simulink model "ballbeam_start"  (R2020b)
settings: Solver=ode4  StartTime=0.0  StopTime=inf  FixedStep=0.002  RelTol=1e-3
model workspace (MAT data in the model file):
  Kc = 14.8792
  Wf = 31.4
  z = 4.0159
undefined symbols (not defined in the file or in its folder): HIL, qc_get_step_size
libraries: quarc_library x3, simulink_extras x1
settings Model: ExtModeTrigDuration=12500  Creator=MLevis  LastModifiedBy=kevin
settings DataIOCC: ReturnWorkspaceOutputs=off
settings DebuggingCC: UnderspecifiedInitializationDetection=Classic  MergeDetectMultiDrivingBlocksExec=none
settings ModelReferenceCC: PropagateSignalLabelsOutOfModel=off
settings SFSimCC: CustomCodeUndefinedFunction=UseInterfaceOnly

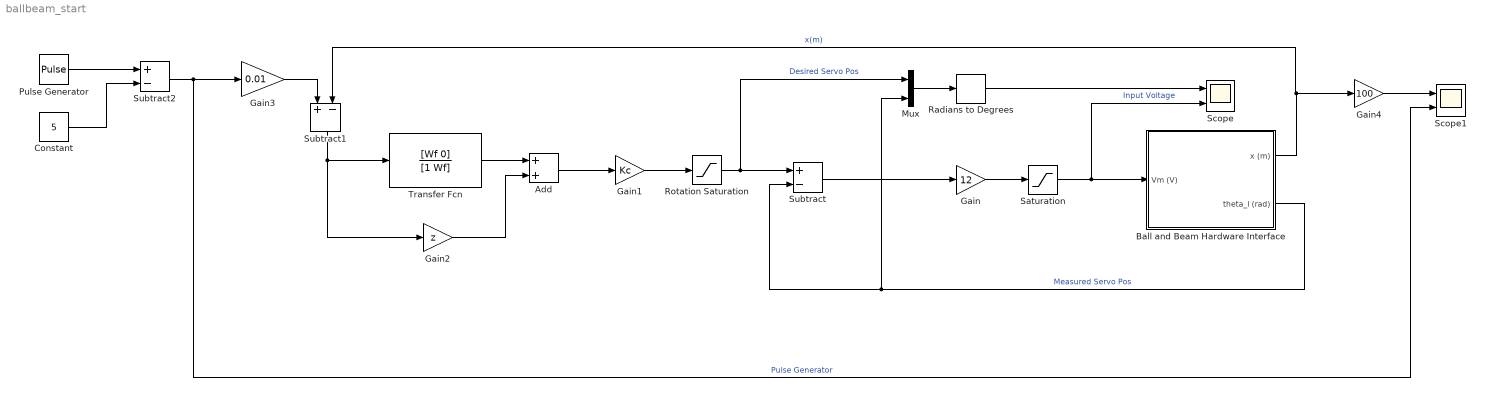
== system ballbeam_start ==
  Add : Sum
  Ball and Beam Hardware Interface : Subsystem
  Constant : Constant  Value=5
  Gain : Gain  Gain=12
  Gain1 : Gain  Gain=Kc
  Gain2 : Gain  Gain=z
  Gain3 : Gain  Gain=0.01
  Gain4 : Gain  Gain=100
  Mux : Mux  Inputs=2
  Pulse Generator : DiscretePulseGenerator  PulseType=Time based  Amplitude=10  Period=10  PulseWidth=50
  Radians to Degrees : simulink_extras/Transformations/Radians to Degrees
  Rotation Saturation : Saturate  UpperLimit=56  LowerLimit=-56
  Saturation : Saturate  UpperLimit=10  LowerLimit=-10
  Scope : Scope  NumInputPorts=2
  Scope1 : Scope  NumInputPorts=2
  Subtract : Sum  Inputs=+-
  Subtract1 : Sum  Inputs=+-
  Subtract2 : Sum  Inputs=+-
  Transfer Fcn : TransferFcn  Numerator=[Wf 0]  Denominator=[1 Wf]
  wires:
  Saturation/1 -> Scope/2, Ball and Beam Hardware Interface/1(Vm (V))  "Input Voltage"
  Gain/1 -> Saturation/1
  Ball and Beam Hardware Interface/2(theta_l (rad)) -> Mux/2, Subtract/2  "Measured Servo Pos"
  Rotation Saturation/1 -> Mux/1, Subtract/1  "Desired Servo Pos"
  Mux/1 -> Radians to Degrees/1
  Radians to Degrees/1 -> Scope/1
  Gain1/1 -> Rotation Saturation/1
  Add/1 -> Gain1/1
  Transfer Fcn/1 -> Add/1
  Gain2/1 -> Add/2
  Subtract1/1 -> Gain2/1, Transfer Fcn/1
  Ball and Beam Hardware Interface/1(x (m)) -> Gain4/1, Subtract1/2  "x(m)"
  Gain3/1 -> Subtract1/1
  Gain4/1 -> Scope1/1
  Constant/1 -> Subtract2/2
  Pulse Generator/1 -> Subtract2/1
  Subtract2/1 -> Scope1/2, Gain3/1  "Pulse Generator"
  Subtract/1 -> Gain/1

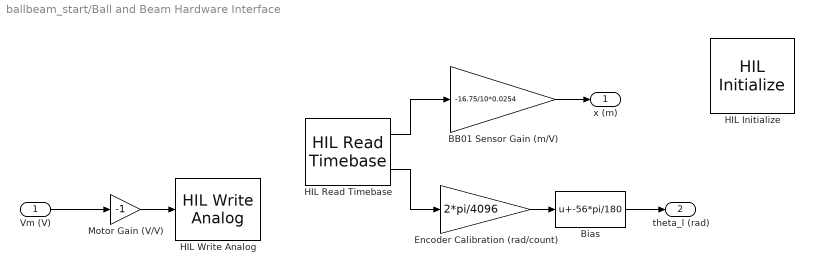
== system ballbeam_start/Ball and Beam Hardware Interface ==
  Vm (V) : Inport
  BB01 Sensor Gain (m/V) : Gain  Gain=-16.75/10*0.0254
  Bias : Bias  Bias=-56*pi/180
  Encoder Calibration (rad/count) : Gain  Gain=2*pi/4096  SaturateOnIntegerOverflow=on  OutDataTypeStr=Inherit: Same as input  ParamDataTypeStr=Inherit: Same as input
  HIL Initialize : quarc_library/Data Acquisition/Generic/Configuration/HIL Initialize  object_name=HIL-1  board_type=q8_usb  board_number=0@tcpip://localhost:18942  board_options=""  exclusive=off  active=on  hardware_clocks=[0:2]  clock_modes=[]  initial_clock_frequencies=[]  set_clock_params_at_start=off  set_clock_params_at_switch_in=off  set_clock_frequencies_at_start=off  set_clock_frequencies_at_switch_in=off  analog_input_channels=[0:7]  analog_input_configurations=[]  analog_input_maximums=10  analog_input_minimums=-10  set_analog_input_params_at_start=on  set_analog_input_params_at_switch_in=off  analog_output_channels=[0:7]  analog_output_maximums=10  analog_output_minimums=-10  initial_analog_outputs=[0]  final_analog_outputs=[0]  watchdog_analog_outputs=0  set_analog_output_params_at_start=on  set_analog_output_params_at_switch_in=off  set_analog_outputs_at_start=on  set_analog_outputs_at_switch_in=off  set_analog_outputs_at_terminate=on  set_analog_outputs_at_switch_out=off  set_analog_outputs_on_watchdog=off  digital_input_channels=[]  digital_output_channels=[0:7]  digital_output_configuration=[]  initial_digital_outputs=[0]  final_digital_outputs=[0]  watchdog_digital_outputs=[0]  set_digital_output_params_at_start=off  set_digital_output_params_at_switch_in=off  set_digital_outputs_at_start=on  set_digital_outputs_at_switch_in=off  set_digital_outputs_at_terminate=on  set_digital_outputs_at_switch_out=off  set_digital_outputs_on_watchdog=off  encoder_channels=[0:7]  quadrature=[4]  encoder_filter_frequency=[]  initial_encoder_counts=[0]  set_encoder_params_at_start=on  set_encoder_params_at_switch_in=off  set_encoder_counts_at_start=on  set_encoder_counts_at_switch_in=off  pwm_channels=[0:7]  pwm_modes=0  pwm_frequency=99.532799999999995e6/4095  pwm_configuration=[0]  pwm_alignment=[0]  pwm_polarity=[1]  pwm_leading_deadband=[0]  pwm_trailing_deadband=[0]  initial_pwm_outputs=[0]  final_pwm_outputs=[0]  watchdog_pwm_outputs=[0]  set_pwm_params_at_start=on  set_pwm_params_at_switch_in=off  set_pwm_outputs_at_start=on  set_pwm_outputs_at_switch_in=off  set_pwm_outputs_at_terminate=on  set_pwm_outputs_at_switch_out=off  set_pwm_outputs_on_watchdog=off  other_output_channels=[]  initial_other_outputs=[]  final_other_outputs=[]  watchdog_other_outputs=[]  set_other_outputs_at_start=off  set_other_outputs_at_switch_in=off  set_other_outputs_at_terminate=off  set_other_outputs_at_switch_out=off  set_other_outputs_on_watchdog=off
  HIL Read Timebase : quarc_library/Data Acquisition/Generic/Timebases/HIL Read Timebase  object_name=HIL-1  clock=0  analog_channels=0  encoder_channels=[0]  digital_channels=[]  other_channels=[]  active=on  vector_output=off  data_type_mode=Inherit via back propagation  encoder_data_type=double  digital_data_type=boolean  overflow_mode=Error on overflow  samples_in_buffer=max(ceil(1/qc_get_step_size), 1)
  HIL Write Analog : quarc_library/Data Acquisition/Generic/Immediate I//O/HIL Write Analog  Tag=unassigned  object_name=HIL-1  channels=0  sample_time=-1  active=on  vector_input=off
  Motor Gain (V/V) : Gain  Gain=-1
  x (m) : Outport  VectorParamsAs1DForOutWhenUnconnected=off
  theta_l (rad) : Outport  Port=2  VectorParamsAs1DForOutWhenUnconnected=off
  wires:
  HIL Read Timebase/2 -> Encoder Calibration (rad/count)/1
  Encoder Calibration (rad/count)/1 -> Bias/1
  HIL Read Timebase/1 -> BB01 Sensor Gain (m/V)/1
  Vm (V)/1 -> Motor Gain (V/V)/1
  Motor Gain (V/V)/1 -> HIL Write Analog/1
  Bias/1 -> theta_l (rad)/1
  BB01 Sensor Gain (m/V)/1 -> x (m)/1
